simulink model "EC_tiempos_servicio"  (R2023b)
settings: Solver=VariableStepAuto  StartTime=0.0  StopTime=25  RelTol=1e-3
undefined symbols (not defined in the file or in its folder): m, n
libraries: simulink x1
settings Model: Creator=anruk  LastModifiedBy=anruk

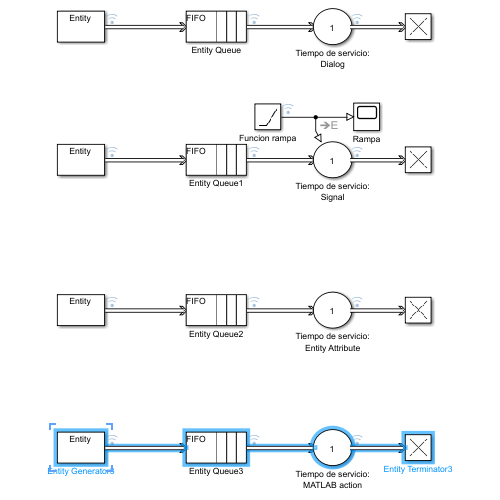
[thumbnail: Simulink's stored preview of the top-level diagram]
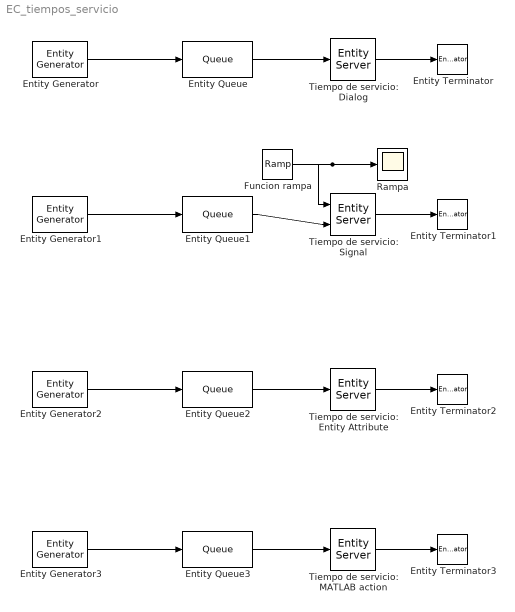
== system EC_tiempos_servicio ==
  Entity Generator : EntityGenerator  OutputPortMessageModes=m  EntityType=Structured  EntityTypeName=Entity
  Entity Generator1 : EntityGenerator  OutputPortMessageModes=m  EntityType=Structured  EntityTypeName=Entity
  Entity Generator2 : EntityGenerator  OutputPortMessageModes=m  AttributeInitialValue=4  EntityType=Structured  EntityTypeName=Entity
  Entity Generator3 : EntityGenerator  OutputPortMessageModes=m  AttributeInitialValue=4  EntityType=Structured  EntityTypeName=Entity
  Entity Queue{,1..3} (4 alike) : Queue  InputPortMessageModes=m  OutputPortMessageModes=m
  Entity Terminator{,1..3} (4 alike) : EntityTerminator  InputPortMessageModes=m
  Funcion rampa : simulink/Sources/Ramp  slope=1  start=0  InitialOutput=0
  Rampa : Scope
  Tiempo de servicio: Dialog : EntityServer  InputPortMessageModes=m  OutputPortMessageModes=m  Capacity=1  ServiceTimeValue=2
  Tiempo de servicio: Entity Attribute : EntityServer  InputPortMessageModes=m  OutputPortMessageModes=m  Capacity=1  ServiceTimeSource=Attribute  ServiceTimeValue=2  ServiceTimeAttributeName=Attribute1
  Tiempo de servicio: MATLAB action : EntityServer  InputPortMessageModes=m  OutputPortMessageModes=m  Capacity=1  ServiceTimeSource=MATLAB action  ServiceTimeValue=2  ServiceTimeAttributeName=Attribute1
  Tiempo de servicio: Signal : EntityServer  InputPortMessageModes=n,m  OutputPortMessageModes=m  Capacity=1  ServiceTimeSource=Signal port  ServiceTimeValue=2
      settings: InputPortMap=u0,u2
  wires:
  Entity Generator/1 -> Entity Queue/1
  Tiempo de servicio: Dialog/1 -> Entity Terminator/1
  Entity Queue/1 -> Tiempo de servicio: Dialog/1
  Entity Queue1/1 -> Tiempo de servicio: Signal/2
  Entity Generator1/1 -> Entity Queue1/1
  Tiempo de servicio: Signal/1 -> Entity Terminator1/1
  Funcion rampa/1 -> Rampa/1, Tiempo de servicio: Signal/1
  Entity Queue2/1 -> Tiempo de servicio: Entity Attribute/1
  Entity Generator2/1 -> Entity Queue2/1
  Tiempo de servicio: Entity Attribute/1 -> Entity Terminator2/1
  Entity Generator3/1 -> Entity Queue3/1
  Tiempo de servicio: MATLAB action/1 -> Entity Terminator3/1
  Entity Queue3/1 -> Tiempo de servicio: MATLAB action/1
